simulink model "IK_corrado"  (R2023b)
settings: Solver=VariableStepAuto  StartTime=0.0  StopTime=15  MaxStep=0.05  RelTol=1e-3
model workspace: external: MAT-File (data not in the file)
libraries: robotcorelib x1, robotmaniplib x1
settings Model: Creator=benit  LastModifiedBy=Savio Del Peschio
settings OptimizationCC: ReuseModelBlockBuffer=off

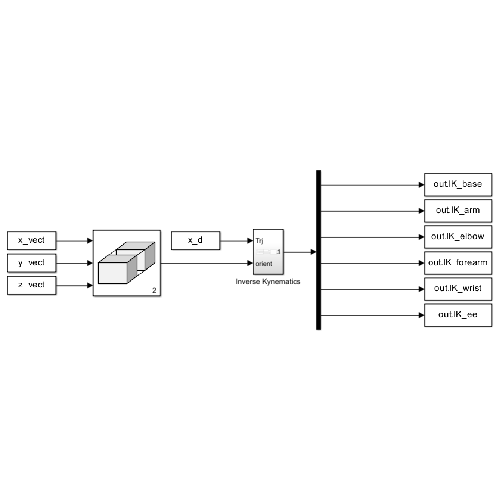
[thumbnail: Simulink's stored preview of the top-level diagram]
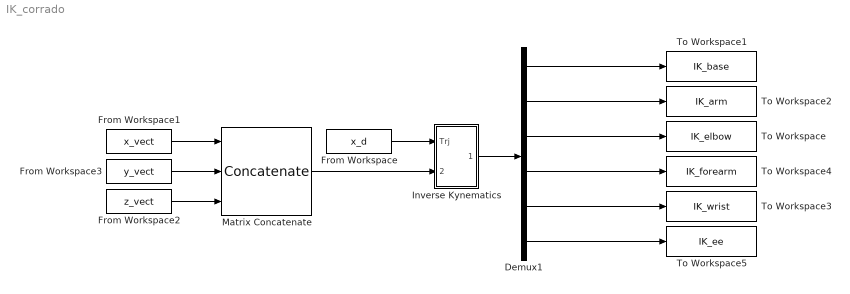
== system IK_corrado ==
  Demux1 : Demux  Outputs=6
  From Workspace : FromWorkspace  VariableName=x_d
  From Workspace1 : FromWorkspace  VariableName=x_vect
  From Workspace2 : FromWorkspace  VariableName=z_vect
  From Workspace3 : FromWorkspace  VariableName=y_vect
  Inverse Kynematics : Subsystem
  Matrix Concatenate : Concatenate  NumInputs=3  Mode=Multidimensional array  ConcatenateDimension=2
  To Workspace : ToWorkspace  VariableName=IK_elbow  SaveFormat=Timeseries  SampleTime=-1
  To Workspace1 : ToWorkspace  VariableName=IK_base  SaveFormat=Timeseries  SampleTime=-1
  To Workspace2 : ToWorkspace  VariableName=IK_arm  SaveFormat=Timeseries  SampleTime=-1
  To Workspace3 : ToWorkspace  VariableName=IK_wrist  SaveFormat=Timeseries  SampleTime=-1
  To Workspace4 : ToWorkspace  VariableName=IK_forearm  SaveFormat=Timeseries  SampleTime=-1
  To Workspace5 : ToWorkspace  VariableName=IK_ee  SaveFormat=Timeseries  SampleTime=-1
  wires:
  Inverse Kynematics/1(Outport) -> Demux1/1
  Demux1/2 -> To Workspace2/1
  Demux1/3 -> To Workspace/1
  Demux1/1 -> To Workspace1/1
  Demux1/5 -> To Workspace3/1
  Demux1/4 -> To Workspace4/1
  From Workspace2/1 -> Matrix Concatenate/3
  From Workspace3/1 -> Matrix Concatenate/2
  From Workspace1/1 -> Matrix Concatenate/1
  Matrix Concatenate/1 -> Inverse Kynematics/2(orient)
  Demux1/6 -> To Workspace5/1
  From Workspace/1 -> Inverse Kynematics/1(Trj)

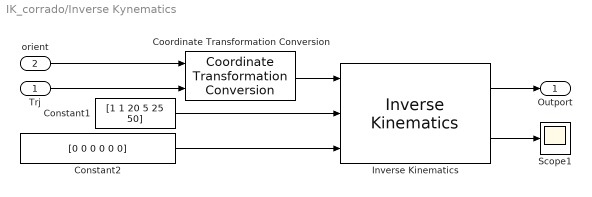
== system IK_corrado/Inverse Kynematics ==
  Trj : Inport
  orient : Inport  Port=2
  Constant1 : Constant  Value=[1 1 20 5 25 50]
  Constant2 : Constant  Value=[0 0 0 0 0 0]
  Coordinate Transformation Conversion : robotcorelib/Coordinate Transformation Conversion  InputRepresentation=Rotation Matrix  InputEulerSequence=ZYX  ShowTrVecInputPort=on  OutputRepresentation=Homogeneous Transformation  OutputEulerSequence=ZYX  ShowTrVecOutputPort=on  SimulateUsing=Interpreted execution
  Inverse Kinematics : robotmaniplib/Inverse Kinematics  RigidBodyTree=corrado  EndEffector=Body6  ShowInfo=on  SolverName=BFGS Gradient Projection  EnforceJointLimits=on  MaxIterations=1500  MaxTime=10  GradientTolerance=1e-7  SolutionTolerance=1e-6  StepTolerance=1e-14  ErrorChangeTolerance=1e-12  UseErrorDamping=on  DampingBias=0.0025  SimulateUsing=Interpreted execution
  Scope1 : Scope
  Outport : Outport
  wires:
  Constant2/1 -> Inverse Kinematics/3
  Constant1/1 -> Inverse Kinematics/2
  Inverse Kinematics/1 -> Outport/1
  Trj/1 -> Coordinate Transformation Conversion/2
  orient/1 -> Coordinate Transformation Conversion/1
  Coordinate Transformation Conversion/1 -> Inverse Kinematics/1
  Inverse Kinematics/2 -> Scope1/1
